simulink model "kick_lowerlimb"  (R2021b)
settings: Solver=FixedStepAuto  StartTime=0.0  StopTime=5  FixedStep=1e-4  RelTol=1e-3  AbsTol=1e-3  EnableMultiTasking=on
values from neighbouring files (symbols this model uses):
  musEnd1 = RN    [runsim.m]
  musEnd2 = RN    [runsim.m]
  musStart1 = -RN    [runsim.m]
  musStart2 = -RN    [runsim.m]
  t1 = 1    [runsim.m]
  t2 = 1.1    [runsim.m]
undefined symbols (not defined in the file or in its folder): intv, param, Param_Mus_MEE, Param_Mus_MEE_hip, Param_Mus_MEE_knee, Param_Mus_MEF, Param_Mus_MEF_hip, Param_Mus_MEF_knee, r, u1, X, Y, Z
libraries: sm_lib x53, Library_mtu_simulink x24, nesl_utility x22
(part 2 of 2)

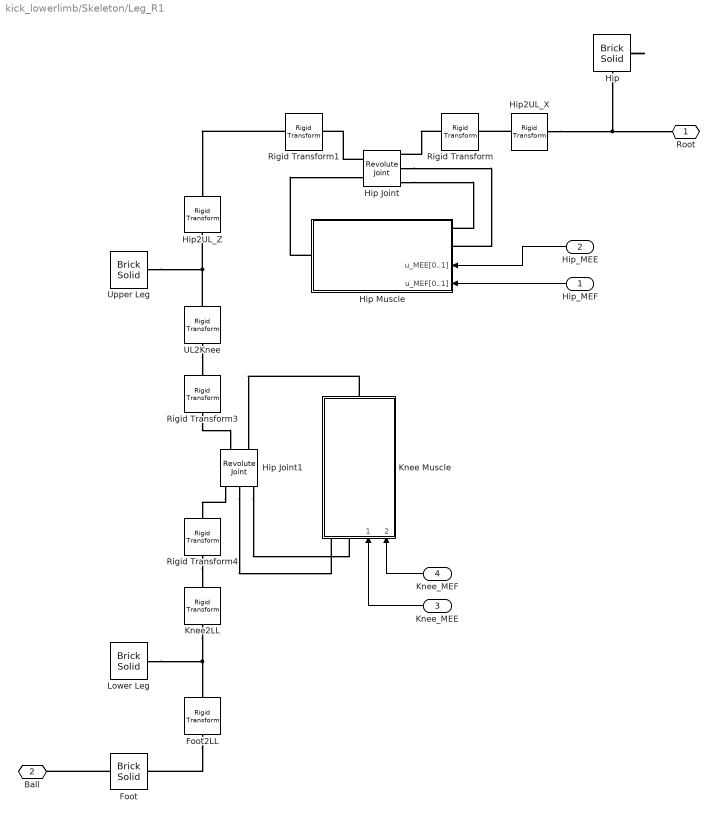
== system kick_lowerlimb/Skeleton/Leg_R1 ==
  Hip_MEF : Inport
  Hip_MEE : Inport  Port=2
  Knee_MEE : Inport  Port=3
  Knee_MEF : Inport  Port=4
  Foot : sm_lib/Body Elements/Brick Solid  GraphicAmbientColor=[0.15 0.15 0.15 1.0]  BasedOnType=Mass  BrickDimensions=param.foot.dim  BrickDimensionUnits=m  CenterOfMass=[0 0 0]  CenterOfMassUnits=m  GraphicDiffuseColor=[0.5 0.5 0.5]  Density=1000  DensityUnits=kg/m^3  DoExposeReferenceFrame=on  GraphicEmissiveColor=[0.0 0.0 0.0 1.0]  ExportEntireGeometry=on  SerializedFrames=<Frames/>  MarkerShape=Sphere  MarkerSize=10  GraphicType=FromGeometry  InertiaType=CalculateFromGeometry  Mass=param.foot.mass  MassUnits=kg  MomentsOfInertia=[1 1 1]  MomentsOfInertiaUnits=kg*m^2  GraphicOpacity=1.0  ProductsOfInertia=[0 0 0]  ProductsOfInertiaUnits=kg*m^2  GraphicShininess=75  GraphicSpecularColor=[0.5 0.5 0.5 1.0]  GraphicVisPropType=SimpleVisualProperties
  Foot2LL : sm_lib/Frames and Transforms/Rigid Transform  TranslationMethod=Cartesian  TranslationStandardOffset=0  TranslationLengthUnit=m  TranslationStandardAxis=+Z  TranslationCartesianOffset=param.ll.pos.foot  TranslationROffset=0  TranslationROffsetUnits=m  TranslationZOffset=0  TranslationZOffsetUnits=m  TranslationThetaOffset=0  TranslationThetaOffsetUnits=deg  RotationMethod=None  RotationAngleUnits=deg  RotationStandardAxis=+Z  RotationAngle=0.0  RotationArbitraryAxis=[0 0 1]  FollAlignAxisA=+X  BaseAlignAxisA=+Y  FollAlignAxisB=+Y  BaseAlignAxisB=+Z  RotationSequenceAxes=FollowerAxes  RotationSequence=XYX  RotationSequenceAngles=[0 0 0]  RotationSequenceAnglesUnits=deg  RotationMatrix=[1 0 0; 0 1 0; 0 0 1]
  Hip : sm_lib/Body Elements/Brick Solid  GraphicAmbientColor=[0.15 0.15 0.15 1.0]  BasedOnType=Mass  BrickDimensions=param.hip.dim  BrickDimensionUnits=m  CenterOfMass=[0 0 0]  CenterOfMassUnits=m  GraphicDiffuseColor=[0.5 0.5 0.5]  Density=1000  DensityUnits=kg/m^3  DoExposeReferenceFrame=on  GraphicEmissiveColor=[0.0 0.0 0.0 1.0]  ExportEntireGeometry=off  SerializedFrames=<Frames/>  MarkerShape=Sphere  MarkerSize=10  GraphicType=FromGeometry  InertiaType=CalculateFromGeometry  Mass=param.hip.mass/2  MassUnits=kg  MomentsOfInertia=[1 1 1]  MomentsOfInertiaUnits=kg*m^2  GraphicOpacity=1.0  ProductsOfInertia=[0 0 0]  ProductsOfInertiaUnits=kg*m^2  GraphicShininess=75  GraphicSpecularColor=[0.5 0.5 0.5 1.0]  GraphicVisPropType=SimpleVisualProperties
  Hip Joint : sm_lib/Joints/Revolute Joint  JointMode=Normal  SenseConstraintForce=off  SenseConstraintForceX=off  SenseConstraintForceY=off  SenseConstraintForceZ=off  SenseConstraintTorque=off  SenseConstraintTorqueX=off  SenseConstraintTorqueY=off  SenseConstraintTorqueZ=off  SenseTotalForce=off  SenseTotalForceX=off  SenseTotalForceY=off  SenseTotalForceZ=off  SenseTotalTorque=off  SenseTotalTorqueX=off  SenseTotalTorqueY=off  SenseTotalTorqueZ=off  CompositeWrenchDir=FollowerOnBase  CompositeWrenchFrame=BaseFrame  EquilibriumPosition=0  EquilibriumPositionUnits=deg  SpringStiffness=0  SpringStiffnessUnits=N*m/deg  DampingCoefficient=0  DampingCoefficientUnits=N*m/(deg/s)  TorqueActuationMode=InputTorque  MotionActuationMode=ComputedMotion  SensePosition=on  SenseVelocity=on  SenseAcceleration=off  SenseTorqueForce=off  SenseLowerLimitTorqueForce=off  SenseUpperLimitTorqueForce=off  LowerLimitSpecify=on  LowerLimitBound=-45  LowerLimitBoundUnits=deg  LowerLimitStiffness=1e4  LowerLimitStiffnessUnits=N*m/deg  LowerLimitDamping=10  LowerLimitDampingUnits=N*m/(deg/s)  LowerLimitTransitionRegionWidth=0.1  LowerLimitTransitionRegionWidthUnits=deg  UpperLimitSpecify=on  UpperLimitBound=90  UpperLimitBoundUnits=deg  UpperLimitStiffness=1e4  UpperLimitStiffnessUnits=N*m/deg  UpperLimitDamping=10  UpperLimitDampingUnits=N*m/(deg/s)  UpperLimitTransitionRegionWidth=0.1  UpperLimitTransitionRegionWidthUnits=deg  PositionTargetSpecify=off  PositionTargetPriority=High  PositionTargetValue=0  PositionTargetValueUnits=deg  VelocityTargetSpecify=off  VelocityTargetPriority=High  VelocityTargetValue=0  VelocityTargetValueUnits=deg/s
  Hip Joint1 : sm_lib/Joints/Revolute Joint  JointMode=Normal  SenseConstraintForce=off  SenseConstraintForceX=off  SenseConstraintForceY=off  SenseConstraintForceZ=off  SenseConstraintTorque=off  SenseConstraintTorqueX=off  SenseConstraintTorqueY=off  SenseConstraintTorqueZ=off  SenseTotalForce=off  SenseTotalForceX=off  SenseTotalForceY=off  SenseTotalForceZ=off  SenseTotalTorque=off  SenseTotalTorqueX=off  SenseTotalTorqueY=off  SenseTotalTorqueZ=off  CompositeWrenchDir=FollowerOnBase  CompositeWrenchFrame=BaseFrame  EquilibriumPosition=0  EquilibriumPositionUnits=deg  SpringStiffness=0  SpringStiffnessUnits=N*m/deg  DampingCoefficient=0  DampingCoefficientUnits=N*m/(deg/s)  TorqueActuationMode=InputTorque  MotionActuationMode=ComputedMotion  SensePosition=on  SenseVelocity=on  SenseAcceleration=off  SenseTorqueForce=off  SenseLowerLimitTorqueForce=off  SenseUpperLimitTorqueForce=off  LowerLimitSpecify=on  LowerLimitBound=-165  LowerLimitBoundUnits=deg  LowerLimitStiffness=1e4  LowerLimitStiffnessUnits=N*m/deg  LowerLimitDamping=10  LowerLimitDampingUnits=N*m/(deg/s)  LowerLimitTransitionRegionWidth=0.1  LowerLimitTransitionRegionWidthUnits=deg  UpperLimitSpecify=on  UpperLimitBound=3  UpperLimitBoundUnits=deg  UpperLimitStiffness=1e4  UpperLimitStiffnessUnits=N*m/deg  UpperLimitDamping=10  UpperLimitDampingUnits=N*m/(deg/s)  UpperLimitTransitionRegionWidth=0.1  UpperLimitTransitionRegionWidthUnits=deg  PositionTargetSpecify=off  PositionTargetPriority=High  PositionTargetValue=0  PositionTargetValueUnits=deg  VelocityTargetSpecify=off  VelocityTargetPriority=High  VelocityTargetValue=0  VelocityTargetValueUnits=deg/s
  Hip Muscle : Subsystem
      settings: PortSchema="{\"entries\":[{\"content\":{\"sides\":[{\"content\":{\"connectorIds\":[\"LConn1\"]},\"type\":\"ConnectorPlacement.EquallySpacedRectSide\",\"uuid\":\"09d485eb-322b-4a2d-b7b4-821800bf0a85\"},{\"content\":{\"connectorIds\":[\"RConn1\",\"RConn2\",\"In1\",\"In2\"],\"side\":\"RIGHT\"},\"type\":\"ConnectorPlacement.EquallySpacedRectSide\",\"uuid\":\"714a60c3-3d51-49b7-818d-6b831f6e3c7a\"},{\"content\":{\"connectorIds\":[],\"side\":\"TOP\"},\"type\":\"ConnectorPlacement.EquallySpacedRectSide\",\"uuid\":\"17f78a34-f772-4722-9987-c43901f4dd6e\"}]},\"type\":\"ConnectorPlacement.EquallySpacedConnector\",\"uuid\":\"fb4f7900-d8a7-436d-9a98-0d4fc98d81d7\"}],\"packageUris\":[\"http://schema.mathworks.com/mf0/Connector/R2020b\"],\"version\":\"1.0\"}"
  Hip2UL_X : sm_lib/Frames and Transforms/Rigid Transform  TranslationMethod=StandardAxis  TranslationStandardOffset=param.hip.pos.ul_x  TranslationLengthUnit=m  TranslationStandardAxis=-X  TranslationCartesianOffset=[0 0 0]  TranslationROffset=0  TranslationROffsetUnits=m  TranslationZOffset=0  TranslationZOffsetUnits=m  TranslationThetaOffset=0  TranslationThetaOffsetUnits=deg  RotationMethod=None  RotationAngleUnits=deg  RotationStandardAxis=+Z  RotationAngle=0.0  RotationArbitraryAxis=[0 0 1]  FollAlignAxisA=+X  BaseAlignAxisA=+Y  FollAlignAxisB=+Y  BaseAlignAxisB=+Z  RotationSequenceAxes=FollowerAxes  RotationSequence=XYX  RotationSequenceAngles=[0 0 0]  RotationSequenceAnglesUnits=deg  RotationMatrix=[1 0 0; 0 1 0; 0 0 1]
  Hip2UL_Z : sm_lib/Frames and Transforms/Rigid Transform  TranslationMethod=StandardAxis  TranslationStandardOffset=param.hip.pos.ul_z  TranslationLengthUnit=m  TranslationStandardAxis=+Z  TranslationCartesianOffset=[0 0 0]  TranslationROffset=0  TranslationROffsetUnits=m  TranslationZOffset=0  TranslationZOffsetUnits=m  TranslationThetaOffset=0  TranslationThetaOffsetUnits=deg  RotationMethod=None  RotationAngleUnits=deg  RotationStandardAxis=+Z  RotationAngle=0.0  RotationArbitraryAxis=[0 0 1]  FollAlignAxisA=+X  BaseAlignAxisA=+Y  FollAlignAxisB=+Y  BaseAlignAxisB=+Z  RotationSequenceAxes=FollowerAxes  RotationSequence=XYX  RotationSequenceAngles=[0 0 0]  RotationSequenceAnglesUnits=deg  RotationMatrix=[1 0 0; 0 1 0; 0 0 1]
  Knee Muscle : Subsystem
      settings: PortSchema="{\"entries\":[{\"content\":{\"sides\":[{\"content\":{\"connectorIds\":[\"LConn1\",\"LConn2\",\"In1\",\"In2\"]},\"type\":\"ConnectorPlacement.EquallySpacedRectSide\",\"uuid\":\"3b044809-3318-4a6d-8aa6-82c54e5fe3cb\"},{\"content\":{\"connectorIds\":[\"RConn1\"],\"side\":\"RIGHT\"},\"type\":\"ConnectorPlacement.EquallySpacedRectSide\",\"uuid\":\"88d11738-42a2-44aa-8fb0-c3ef05d80cd7\"},{\"content\":{\"connectorIds\":[],\"side\":\"TOP\"},\"type\":\"ConnectorPlacement.EquallySpacedRectSide\",\"uuid\":\"f463f2d8-c609-4ddb-8314-070b29d257df\"}]},\"type\":\"ConnectorPlacement.EquallySpacedConnector\",\"uuid\":\"4bbd78e6-9d91-4575-bf34-482a08640315\"}],\"packageUris\":[\"http://schema.mathworks.com/mf0/Connector/R2020b\"],\"version\":\"1.0\"}"
  Knee2LL : sm_lib/Frames and Transforms/Rigid Transform  TranslationMethod=Cartesian  TranslationStandardOffset=0  TranslationLengthUnit=m  TranslationStandardAxis=+Z  TranslationCartesianOffset=param.ll.pos.knee  TranslationROffset=0  TranslationROffsetUnits=m  TranslationZOffset=0  TranslationZOffsetUnits=m  TranslationThetaOffset=0  TranslationThetaOffsetUnits=deg  RotationMethod=None  RotationAngleUnits=deg  RotationStandardAxis=+Z  RotationAngle=0.0  RotationArbitraryAxis=[0 0 1]  FollAlignAxisA=+X  BaseAlignAxisA=+Y  FollAlignAxisB=+Y  BaseAlignAxisB=+Z  RotationSequenceAxes=FollowerAxes  RotationSequence=XYX  RotationSequenceAngles=[0 0 0]  RotationSequenceAnglesUnits=deg  RotationMatrix=[1 0 0; 0 1 0; 0 0 1]
  Lower Leg : sm_lib/Body Elements/Brick Solid  GraphicAmbientColor=[0.15 0.15 0.15 1.0]  BasedOnType=Mass  BrickDimensions=param.ll.dim  BrickDimensionUnits=m  CenterOfMass=[0 0 0]  CenterOfMassUnits=m  GraphicDiffuseColor=[0.2 0.2 1.0]  Density=1000  DensityUnits=kg/m^3  DoExposeReferenceFrame=on  GraphicEmissiveColor=[0.0 0.0 0.0 1.0]  ExportEntireGeometry=off  SerializedFrames=<Frames/>  MarkerShape=Sphere  MarkerSize=10  GraphicType=FromGeometry  InertiaType=CalculateFromGeometry  Mass=param.ll.mass  MassUnits=kg  MomentsOfInertia=[1 1 1]  MomentsOfInertiaUnits=kg*m^2  GraphicOpacity=1.0  ProductsOfInertia=[0 0 0]  ProductsOfInertiaUnits=kg*m^2  GraphicShininess=75  GraphicSpecularColor=[0.5 0.5 0.5 1.0]  GraphicVisPropType=SimpleVisualProperties
  Rigid Transform : sm_lib/Frames and Transforms/Rigid Transform  TranslationMethod=None  TranslationStandardOffset=0  TranslationLengthUnit=m  TranslationStandardAxis=+Z  TranslationCartesianOffset=[0 0 0]  TranslationROffset=0  TranslationROffsetUnits=m  TranslationZOffset=0  TranslationZOffsetUnits=m  TranslationThetaOffset=0  TranslationThetaOffsetUnits=deg  RotationMethod=StandardAxis  RotationAngleUnits=deg  RotationStandardAxis=+Y  RotationAngle=90  RotationArbitraryAxis=[0 0 1]  FollAlignAxisA=+X  BaseAlignAxisA=+Y  FollAlignAxisB=+Y  BaseAlignAxisB=+Z  RotationSequenceAxes=FollowerAxes  RotationSequence=XYX  RotationSequenceAngles=[0 0 0]  RotationSequenceAnglesUnits=deg  RotationMatrix=[1 0 0; 0 1 0; 0 0 1]
  Rigid Transform1 : sm_lib/Frames and Transforms/Rigid Transform  TranslationMethod=None  TranslationStandardOffset=0  TranslationLengthUnit=m  TranslationStandardAxis=+Z  TranslationCartesianOffset=[0 0 0]  TranslationROffset=0  TranslationROffsetUnits=m  TranslationZOffset=0  TranslationZOffsetUnits=m  TranslationThetaOffset=0  TranslationThetaOffsetUnits=deg  RotationMethod=StandardAxis  RotationAngleUnits=deg  RotationStandardAxis=-Y  RotationAngle=90  RotationArbitraryAxis=[0 0 1]  FollAlignAxisA=+X  BaseAlignAxisA=+Y  FollAlignAxisB=+Y  BaseAlignAxisB=+Z  RotationSequenceAxes=FollowerAxes  RotationSequence=XYX  RotationSequenceAngles=[0 0 0]  RotationSequenceAnglesUnits=deg  RotationMatrix=[1 0 0; 0 1 0; 0 0 1]
  Rigid Transform3 : sm_lib/Frames and Transforms/Rigid Transform  TranslationMethod=None  TranslationStandardOffset=0  TranslationLengthUnit=m  TranslationStandardAxis=+Z  TranslationCartesianOffset=[0 0 0]  TranslationROffset=0  TranslationROffsetUnits=m  TranslationZOffset=0  TranslationZOffsetUnits=m  TranslationThetaOffset=0  TranslationThetaOffsetUnits=deg  RotationMethod=StandardAxis  RotationAngleUnits=deg  RotationStandardAxis=+Y  RotationAngle=90  RotationArbitraryAxis=[0 0 1]  FollAlignAxisA=+X  BaseAlignAxisA=+Y  FollAlignAxisB=+Y  BaseAlignAxisB=+Z  RotationSequenceAxes=FollowerAxes  RotationSequence=XYX  RotationSequenceAngles=[0 0 0]  RotationSequenceAnglesUnits=deg  RotationMatrix=[1 0 0; 0 1 0; 0 0 1]
  Rigid Transform4 : sm_lib/Frames and Transforms/Rigid Transform  TranslationMethod=None  TranslationStandardOffset=0  TranslationLengthUnit=m  TranslationStandardAxis=+Z  TranslationCartesianOffset=[0 0 0]  TranslationROffset=0  TranslationROffsetUnits=m  TranslationZOffset=0  TranslationZOffsetUnits=m  TranslationThetaOffset=0  TranslationThetaOffsetUnits=deg  RotationMethod=StandardAxis  RotationAngleUnits=deg  RotationStandardAxis=-Y  RotationAngle=90  RotationArbitraryAxis=[0 0 1]  FollAlignAxisA=+X  BaseAlignAxisA=+Y  FollAlignAxisB=+Y  BaseAlignAxisB=+Z  RotationSequenceAxes=FollowerAxes  RotationSequence=XYX  RotationSequenceAngles=[0 0 0]  RotationSequenceAnglesUnits=deg  RotationMatrix=[1 0 0; 0 1 0; 0 0 1]
  UL2Knee : sm_lib/Frames and Transforms/Rigid Transform  TranslationMethod=Cartesian  TranslationStandardOffset=0  TranslationLengthUnit=m  TranslationStandardAxis=+Z  TranslationCartesianOffset=param.ul.pos.knee  TranslationROffset=0  TranslationROffsetUnits=m  TranslationZOffset=0  TranslationZOffsetUnits=m  TranslationThetaOffset=0  TranslationThetaOffsetUnits=deg  RotationMethod=None  RotationAngleUnits=deg  RotationStandardAxis=+Z  RotationAngle=0.0  RotationArbitraryAxis=[0 0 1]  FollAlignAxisA=+X  BaseAlignAxisA=+Y  FollAlignAxisB=+Y  BaseAlignAxisB=+Z  RotationSequenceAxes=FollowerAxes  RotationSequence=XYX  RotationSequenceAngles=[0 0 0]  RotationSequenceAnglesUnits=deg  RotationMatrix=[1 0 0; 0 1 0; 0 0 1]
  Upper Leg : sm_lib/Body Elements/Brick Solid  GraphicAmbientColor=[0.15 0.15 0.15 1.0]  BasedOnType=Mass  BrickDimensions=param.ul.dim  BrickDimensionUnits=m  CenterOfMass=[0 0 0]  CenterOfMassUnits=m  GraphicDiffuseColor=[0.5 0.5 0.5]  Density=1000  DensityUnits=kg/m^3  DoExposeReferenceFrame=on  GraphicEmissiveColor=[0.0 0.0 0.0 1.0]  ExportEntireGeometry=off  SerializedFrames=<Frames/>  MarkerShape=Sphere  MarkerSize=10  GraphicType=FromGeometry  InertiaType=CalculateFromGeometry  Mass=param.ul.mass  MassUnits=kg  MomentsOfInertia=[1 1 1]  MomentsOfInertiaUnits=kg*m^2  GraphicOpacity=1.0  ProductsOfInertia=[0 0 0]  ProductsOfInertiaUnits=kg*m^2  GraphicShininess=75  GraphicSpecularColor=[0.5 0.5 0.5 1.0]  GraphicVisPropType=SimpleVisualProperties
  Root : PMIOPort  Side=Left
  Ball : PMIOPort  Port=2  Side=Right
  wires:
  Hip_MEF/1 -> Hip Muscle/2(u_MEF[0..1])
  Hip_MEE/1 -> Hip Muscle/1(u_MEE[0..1])
  Knee_MEE/1 -> Knee Muscle/1(u_MEE[0..1])
  Knee_MEF/1 -> Knee Muscle/2(u_MEF[0..1])
  connections:
  Lower Leg/RConn1 -- Knee2LL/RConn1 -- Foot2LL/LConn1
  Foot2LL/RConn1 -- Foot/RConn1
  UL2Knee/LConn1 -- Upper Leg/RConn1 -- Hip2UL_Z/RConn1
  Hip/RConn1 -- Root/RConn1 -- Hip2UL_X/LConn1
  Rigid Transform/LConn1 -- Hip Joint/RConn1
  Hip Joint/LConn1 -- Rigid Transform1/RConn1
  Hip2UL_X/RConn1 -- Rigid Transform/RConn1
  UL2Knee/RConn1 -- Rigid Transform3/LConn1
  Rigid Transform3/RConn1 -- Hip Joint1/LConn1
  Hip Joint1/RConn1 -- Rigid Transform4/LConn1
  Rigid Transform4/RConn1 -- Knee2LL/LConn1
  Foot/LConn1 -- Ball/RConn1
  Hip Joint/RConn2 -- Hip Muscle/RConn2
  Rigid Transform1/LConn1 -- Hip2UL_Z/LConn1
  Hip Joint/RConn3 -- Hip Muscle/RConn1
  Hip Muscle/LConn1 -- Hip Joint/LConn2
  Hip Joint1/RConn2 -- Knee Muscle/LConn1
  Knee Muscle/RConn1 -- Hip Joint1/LConn2
  Hip Joint1/RConn3 -- Knee Muscle/LConn2

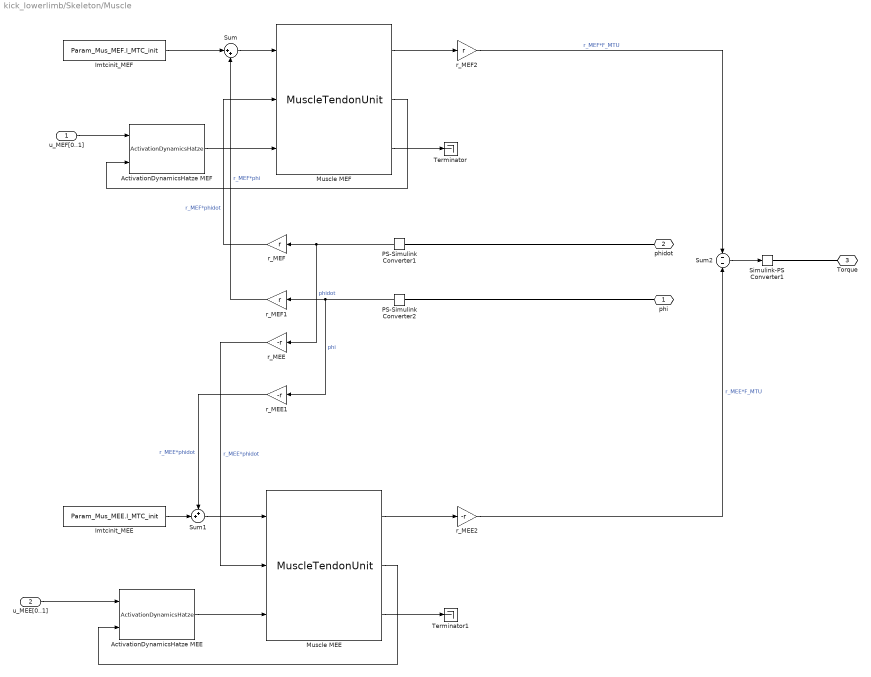
== system kick_lowerlimb/Skeleton/Muscle ==
  u_MEF[0..1] : Inport
  u_MEE[0..1] : Inport  Port=2
  ActivationDynamicsHatze MEE : Library_mtu_simulink/ActivationDynamicsHatze  Act_Param=Param_Mus_MEE.ActDyn  Mus_Param=Param_Mus_MEE
  ActivationDynamicsHatze MEF : Library_mtu_simulink/ActivationDynamicsHatze  Act_Param=Param_Mus_MEF.ActDyn  Mus_Param=Param_Mus_MEF
  Imtcinit_MEE : Constant  Value=Param_Mus_MEE.l_MTC_init
  Imtcinit_MEF : Constant  Value=Param_Mus_MEF.l_MTC_init
  Muscle MEE : Library_mtu_simulink/MuscleTendonUnit  Mus_Param=Param_Mus_MEE
  Muscle MEF : Library_mtu_simulink/MuscleTendonUnit  Mus_Param=Param_Mus_MEF
  PS-Simulink Converter1 : nesl_utility/PS-Simulink Converter  PhysicalDomain=network_engine_domain  SubClassName=ps_output  LeftPortType=input  RightPortType=output  PseudoPeriodic=off  Frequencies=[]  Unit=inherit  AffineConversion=off
      settings: SourceProductBaseCode=PW,SS
  PS-Simulink Converter2 : nesl_utility/PS-Simulink Converter  PhysicalDomain=network_engine_domain  SubClassName=ps_output  LeftPortType=input  RightPortType=output  PseudoPeriodic=off  Frequencies=[]  Unit=inherit  AffineConversion=off
      settings: SourceProductBaseCode=PW,SS
  Simulink-PS Converter1 : nesl_utility/Simulink-PS Converter  PhysicalDomain=network_engine_domain  SubClassName=ps_input  LeftPortType=input  RightPortType=output  PseudoPeriodic=off  Frequencies=[]  NoiseDistribution=none  NoiseParameters=[]  Unit=1  AffineConversion=off  FilteringAndDerivatives=provide  SimscapeFilterOrder=1  InputFilterTimeConstant=0.001  UdotUserProvided=0
      settings: SourceProductBaseCode=PW,SS
  Sum : Sum  Inputs=|++
  Sum1 : Sum  Inputs=++|
  Sum2 : Sum  Inputs=--
  Terminator : Terminator
  Terminator1 : Terminator
  r_MEE : Gain  Gain=-r
  r_MEE1 : Gain  Gain=-r
  r_MEE2 : Gain  Gain=-r
  r_MEF : Gain  Gain=r
  r_MEF1 : Gain  Gain=r
  r_MEF2 : Gain  Gain=r
  phi : PMIOPort  Side=Left
  phidot : PMIOPort  Port=2  Side=Left
  Torque : PMIOPort  Port=3  Side=Right
  wires:
  r_MEE/1 -> Muscle MEE/2  "r_MEE*phidot"
  Imtcinit_MEE/1 -> Sum1/2
  ActivationDynamicsHatze MEF/1 -> Muscle MEF/3
  PS-Simulink Converter2/1 -> r_MEF1/1, r_MEE1/1  "phi"
  r_MEE2/1 -> Sum2/2  "r_MEE*F_MTU"
  u_MEF[0..1]/1 -> ActivationDynamicsHatze MEF/1
  Muscle MEF/3 -> Terminator/1
  r_MEF/1 -> Muscle MEF/2  "r_MEF*phidot"
  Sum/1 -> Muscle MEF/1
  Muscle MEE/1 -> r_MEE2/1
  r_MEE1/1 -> Sum1/1  "r_MEE*phidot"
  r_MEF1/1 -> Sum/2  "r_MEF*phi"
  u_MEE[0..1]/1 -> ActivationDynamicsHatze MEE/1
  Sum2/1 -> Simulink-PS Converter1/1
  Sum1/1 -> Muscle MEE/1
  Imtcinit_MEF/1 -> Sum/1
  PS-Simulink Converter1/1 -> r_MEF/1, r_MEE/1  "phidot"
  ActivationDynamicsHatze MEE/1 -> Muscle MEE/3
  Muscle MEE/2 -> ActivationDynamicsHatze MEE/2
  Muscle MEE/3 -> Terminator1/1
  Muscle MEF/1 -> r_MEF2/1
  Muscle MEF/2 -> ActivationDynamicsHatze MEF/2
  r_MEF2/1 -> Sum2/1  "r_MEF*F_MTU"
  connections:
  Torque/RConn1 -- Simulink-PS Converter1/RConn1
  PS-Simulink Converter2/LConn1 -- phi/RConn1
  PS-Simulink Converter1/LConn1 -- phidot/RConn1

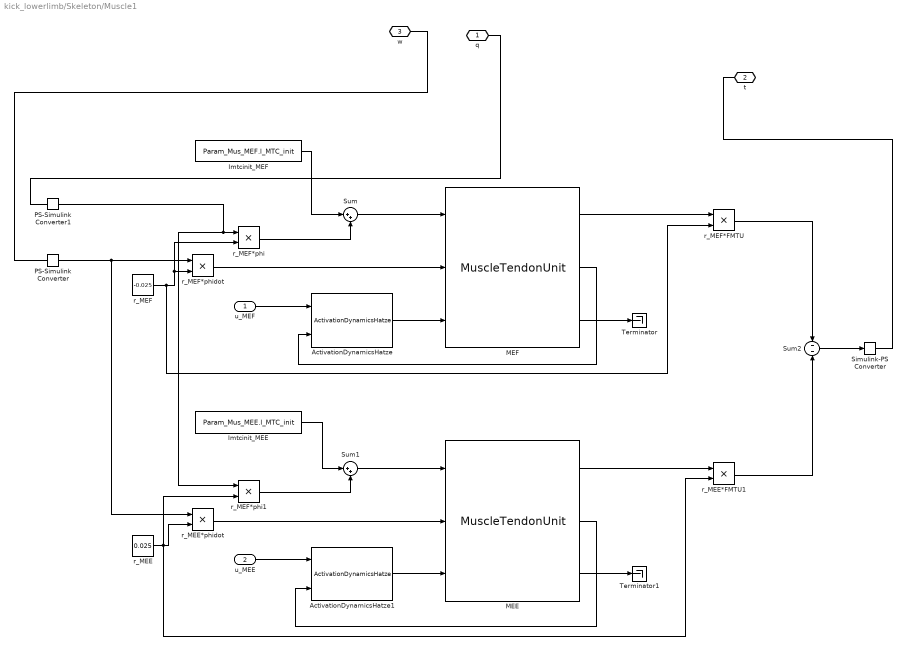
== system kick_lowerlimb/Skeleton/Muscle1 ==
  u_MEF : Inport
  u_MEE : Inport  Port=2
  ActivationDynamicsHatze : Library_mtu_simulink/ActivationDynamicsHatze  Act_Param=Param_Mus_MEF.ActDyn  Mus_Param=Param_Mus_MEF
  ActivationDynamicsHatze1 : Library_mtu_simulink/ActivationDynamicsHatze  Act_Param=Param_Mus_MEE.ActDyn  Mus_Param=Param_Mus_MEE
  Imtcinit_MEE : Constant  Value=Param_Mus_MEE.l_MTC_init
  Imtcinit_MEF : Constant  Value=Param_Mus_MEF.l_MTC_init
  MEE : Library_mtu_simulink/MuscleTendonUnit  Mus_Param=Param_Mus_MEE
  MEF : Library_mtu_simulink/MuscleTendonUnit  Mus_Param=Param_Mus_MEF
  PS-Simulink Converter : nesl_utility/PS-Simulink Converter  PhysicalDomain=network_engine_domain  SubClassName=ps_output  LeftPortType=input  RightPortType=output  PseudoPeriodic=off  Frequencies=[]  Unit=inherit  AffineConversion=off
      settings: SourceProductBaseCode=PW,SS
  PS-Simulink Converter1 : nesl_utility/PS-Simulink Converter  PhysicalDomain=network_engine_domain  SubClassName=ps_output  LeftPortType=input  RightPortType=output  PseudoPeriodic=off  Frequencies=[]  Unit=inherit  AffineConversion=off
      settings: SourceProductBaseCode=PW,SS
  Simulink-PS Converter : nesl_utility/Simulink-PS Converter  PhysicalDomain=network_engine_domain  SubClassName=ps_input  LeftPortType=input  RightPortType=output  PseudoPeriodic=off  Frequencies=[]  NoiseDistribution=none  NoiseParameters=[]  Unit=1  AffineConversion=off  FilteringAndDerivatives=provide  SimscapeFilterOrder=1  InputFilterTimeConstant=0.001  UdotUserProvided=0
      settings: SourceProductBaseCode=PW,SS
  Sum : Sum  Inputs=|++
  Sum1 : Sum  Inputs=|++
  Sum2 : Sum  Inputs=--
  Terminator : Terminator
  Terminator1 : Terminator
  r_MEE : Constant  Value=0.025
  r_MEE*FMTU1 : Product
  r_MEE*phidot : Product
  r_MEF : Constant  Value=-0.025
  r_MEF*FMTU : Product
  r_MEF*phi : Product
  r_MEF*phi1 : Product
  r_MEF*phidot : Product
  q : PMIOPort  Side=Left
  t : PMIOPort  Port=2  Side=Right
  w : PMIOPort  Port=3  Side=Left
  wires:
  r_MEE*FMTU1/1 -> Sum2/2
  r_MEF*FMTU/1 -> Sum2/1
  MEF/3 -> Terminator/1
  r_MEE*phidot/1 -> MEE/2
  Sum2/1 -> Simulink-PS Converter/1
  PS-Simulink Converter1/1 -> r_MEF*phi1/1, r_MEF*phi/1
  PS-Simulink Converter/1 -> r_MEE*phidot/1, r_MEF*phidot/1
  r_MEE/1 -> r_MEE*FMTU1/2, r_MEF*phi1/2, r_MEE*phidot/2
  MEE/2 -> ActivationDynamicsHatze1/2
  Sum/1 -> MEF/1
  r_MEF*phi1/1 -> Sum1/2
  Imtcinit_MEE/1 -> Sum1/1
  MEE/3 -> Terminator1/1
  Imtcinit_MEF/1 -> Sum/1
  u_MEE/1 -> ActivationDynamicsHatze1/1
  r_MEF/1 -> r_MEF*FMTU/2, r_MEF*phi/2, r_MEF*phidot/2
  u_MEF/1 -> ActivationDynamicsHatze/1
  Sum1/1 -> MEE/1
  MEF/1 -> r_MEF*FMTU/1
  ActivationDynamicsHatze1/1 -> MEE/3
  r_MEF*phidot/1 -> MEF/2
  r_MEF*phi/1 -> Sum/2
  MEE/1 -> r_MEE*FMTU1/1
  MEF/2 -> ActivationDynamicsHatze/2
  ActivationDynamicsHatze/1 -> MEF/3
  connections:
  PS-Simulink Converter1/LConn1 -- q/RConn1
  Simulink-PS Converter/RConn1 -- t/RConn1
  PS-Simulink Converter/LConn1 -- w/RConn1

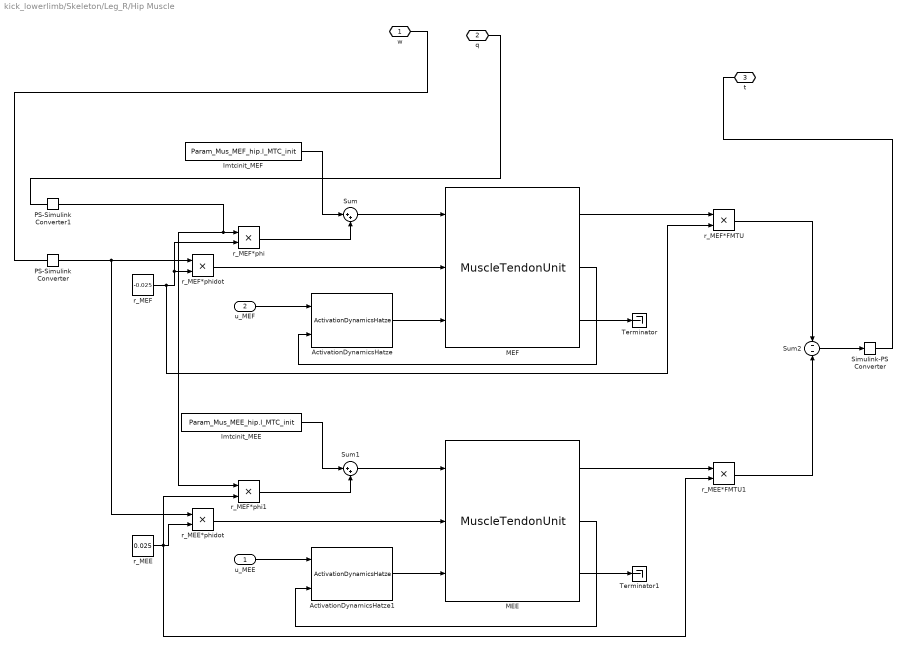
== system kick_lowerlimb/Skeleton/Leg_R/Hip Muscle ==
  u_MEE : Inport
  u_MEF : Inport  Port=2
  ActivationDynamicsHatze : Library_mtu_simulink/ActivationDynamicsHatze  Act_Param=Param_Mus_MEF_hip.ActDyn  Mus_Param=Param_Mus_MEF_hip
  ActivationDynamicsHatze1 : Library_mtu_simulink/ActivationDynamicsHatze  Act_Param=Param_Mus_MEE_hip.ActDyn  Mus_Param=Param_Mus_MEE_hip
  Imtcinit_MEE : Constant  Value=Param_Mus_MEE_hip.l_MTC_init
  Imtcinit_MEF : Constant  Value=Param_Mus_MEF_hip.l_MTC_init
  MEE : Library_mtu_simulink/MuscleTendonUnit  Mus_Param=Param_Mus_MEE_hip
  MEF : Library_mtu_simulink/MuscleTendonUnit  Mus_Param=Param_Mus_MEF_hip
  PS-Simulink Converter : nesl_utility/PS-Simulink Converter  PhysicalDomain=network_engine_domain  SubClassName=ps_output  LeftPortType=input  RightPortType=output  PseudoPeriodic=off  Frequencies=[]  Unit=inherit  AffineConversion=off
      settings: SourceProductBaseCode=PW,SS
  PS-Simulink Converter1 : nesl_utility/PS-Simulink Converter  PhysicalDomain=network_engine_domain  SubClassName=ps_output  LeftPortType=input  RightPortType=output  PseudoPeriodic=off  Frequencies=[]  Unit=inherit  AffineConversion=off
      settings: SourceProductBaseCode=PW,SS
  Simulink-PS Converter : nesl_utility/Simulink-PS Converter  PhysicalDomain=network_engine_domain  SubClassName=ps_input  LeftPortType=input  RightPortType=output  PseudoPeriodic=off  Frequencies=[]  NoiseDistribution=none  NoiseParameters=[]  Unit=1  AffineConversion=off  FilteringAndDerivatives=provide  SimscapeFilterOrder=1  InputFilterTimeConstant=0.001  UdotUserProvided=0
      settings: SourceProductBaseCode=PW,SS
  Sum : Sum  Inputs=|++
  Sum1 : Sum  Inputs=|++
  Sum2 : Sum  Inputs=--
  Terminator : Terminator
  Terminator1 : Terminator
  r_MEE : Constant  Value=0.025
  r_MEE*FMTU1 : Product
  r_MEE*phidot : Product
  r_MEF : Constant  Value=-0.025
  r_MEF*FMTU : Product
  r_MEF*phi : Product
  r_MEF*phi1 : Product
  r_MEF*phidot : Product
  w : PMIOPort  Side=Left
  q : PMIOPort  Port=2  Side=Left
  t : PMIOPort  Port=3  Side=Right
  wires:
  r_MEE*FMTU1/1 -> Sum2/2
  r_MEF*FMTU/1 -> Sum2/1
  MEF/3 -> Terminator/1
  r_MEE*phidot/1 -> MEE/2
  Sum2/1 -> Simulink-PS Converter/1
  PS-Simulink Converter1/1 -> r_MEF*phi1/1, r_MEF*phi/1
  PS-Simulink Converter/1 -> r_MEE*phidot/1, r_MEF*phidot/1
  r_MEE/1 -> r_MEE*FMTU1/2, r_MEF*phi1/2, r_MEE*phidot/2
  MEE/2 -> ActivationDynamicsHatze1/2
  Sum/1 -> MEF/1
  r_MEF*phi1/1 -> Sum1/2
  Imtcinit_MEE/1 -> Sum1/1
  MEE/3 -> Terminator1/1
  Imtcinit_MEF/1 -> Sum/1
  u_MEE/1 -> ActivationDynamicsHatze1/1
  r_MEF/1 -> r_MEF*FMTU/2, r_MEF*phi/2, r_MEF*phidot/2
  u_MEF/1 -> ActivationDynamicsHatze/1
  Sum1/1 -> MEE/1
  MEF/1 -> r_MEF*FMTU/1
  ActivationDynamicsHatze1/1 -> MEE/3
  r_MEF*phidot/1 -> MEF/2
  r_MEF*phi/1 -> Sum/2
  MEE/1 -> r_MEE*FMTU1/1
  MEF/2 -> ActivationDynamicsHatze/2
  ActivationDynamicsHatze/1 -> MEF/3
  connections:
  PS-Simulink Converter1/LConn1 -- q/RConn1
  Simulink-PS Converter/RConn1 -- t/RConn1
  PS-Simulink Converter/LConn1 -- w/RConn1

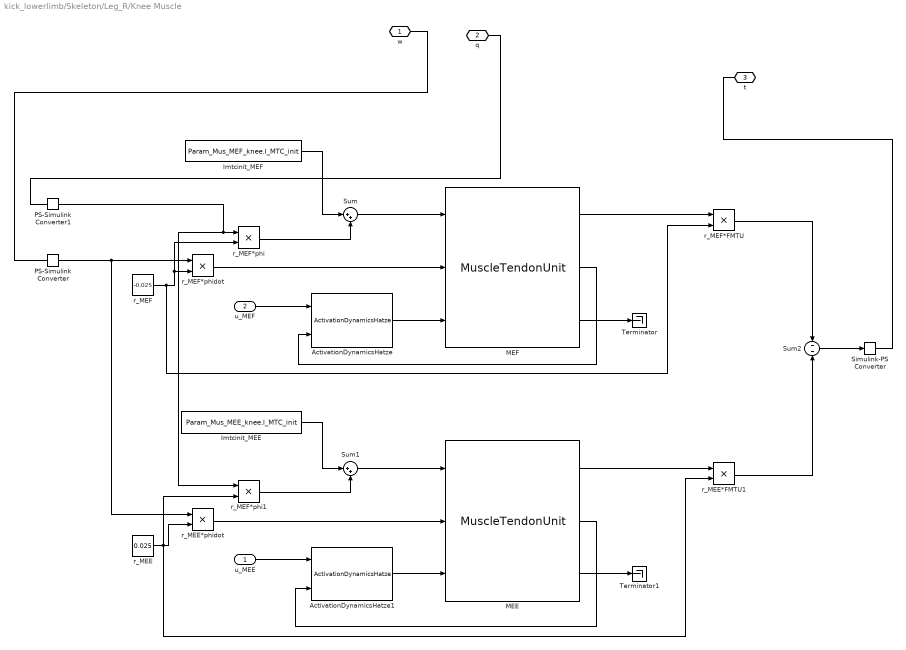
== system kick_lowerlimb/Skeleton/Leg_R/Knee Muscle ==
  u_MEE : Inport
  u_MEF : Inport  Port=2
  ActivationDynamicsHatze : Library_mtu_simulink/ActivationDynamicsHatze  Act_Param=Param_Mus_MEF_knee.ActDyn  Mus_Param=Param_Mus_MEF_knee
  ActivationDynamicsHatze1 : Library_mtu_simulink/ActivationDynamicsHatze  Act_Param=Param_Mus_MEE_knee.ActDyn  Mus_Param=Param_Mus_MEE_knee
  Imtcinit_MEE : Constant  Value=Param_Mus_MEE_knee.l_MTC_init
  Imtcinit_MEF : Constant  Value=Param_Mus_MEF_knee.l_MTC_init
  MEE : Library_mtu_simulink/MuscleTendonUnit  Mus_Param=Param_Mus_MEE_knee
  MEF : Library_mtu_simulink/MuscleTendonUnit  Mus_Param=Param_Mus_MEF_knee
  PS-Simulink Converter : nesl_utility/PS-Simulink Converter  PhysicalDomain=network_engine_domain  SubClassName=ps_output  LeftPortType=input  RightPortType=output  PseudoPeriodic=off  Frequencies=[]  Unit=inherit  AffineConversion=off
      settings: SourceProductBaseCode=PW,SS
  PS-Simulink Converter1 : nesl_utility/PS-Simulink Converter  PhysicalDomain=network_engine_domain  SubClassName=ps_output  LeftPortType=input  RightPortType=output  PseudoPeriodic=off  Frequencies=[]  Unit=inherit  AffineConversion=off
      settings: SourceProductBaseCode=PW,SS
  Simulink-PS Converter : nesl_utility/Simulink-PS Converter  PhysicalDomain=network_engine_domain  SubClassName=ps_input  LeftPortType=input  RightPortType=output  PseudoPeriodic=off  Frequencies=[]  NoiseDistribution=none  NoiseParameters=[]  Unit=1  AffineConversion=off  FilteringAndDerivatives=provide  SimscapeFilterOrder=1  InputFilterTimeConstant=0.001  UdotUserProvided=0
      settings: SourceProductBaseCode=PW,SS
  Sum : Sum  Inputs=|++
  Sum1 : Sum  Inputs=|++
  Sum2 : Sum  Inputs=--
  Terminator : Terminator
  Terminator1 : Terminator
  r_MEE : Constant  Value=0.025
  r_MEE*FMTU1 : Product
  r_MEE*phidot : Product
  r_MEF : Constant  Value=-0.025
  r_MEF*FMTU : Product
  r_MEF*phi : Product
  r_MEF*phi1 : Product
  r_MEF*phidot : Product
  w : PMIOPort  Side=Left
  q : PMIOPort  Port=2  Side=Left
  t : PMIOPort  Port=3  Side=Right
  wires:
  r_MEE*FMTU1/1 -> Sum2/2
  r_MEF*FMTU/1 -> Sum2/1
  MEF/3 -> Terminator/1
  r_MEE*phidot/1 -> MEE/2
  Sum2/1 -> Simulink-PS Converter/1
  PS-Simulink Converter1/1 -> r_MEF*phi1/1, r_MEF*phi/1
  PS-Simulink Converter/1 -> r_MEE*phidot/1, r_MEF*phidot/1
  r_MEE/1 -> r_MEE*FMTU1/2, r_MEF*phi1/2, r_MEE*phidot/2
  MEE/2 -> ActivationDynamicsHatze1/2
  Sum/1 -> MEF/1
  r_MEF*phi1/1 -> Sum1/2
  Imtcinit_MEE/1 -> Sum1/1
  MEE/3 -> Terminator1/1
  Imtcinit_MEF/1 -> Sum/1
  u_MEE/1 -> ActivationDynamicsHatze1/1
  r_MEF/1 -> r_MEF*FMTU/2, r_MEF*phi/2, r_MEF*phidot/2
  u_MEF/1 -> ActivationDynamicsHatze/1
  Sum1/1 -> MEE/1
  MEF/1 -> r_MEF*FMTU/1
  ActivationDynamicsHatze1/1 -> MEE/3
  r_MEF*phidot/1 -> MEF/2
  r_MEF*phi/1 -> Sum/2
  MEE/1 -> r_MEE*FMTU1/1
  MEF/2 -> ActivationDynamicsHatze/2
  ActivationDynamicsHatze/1 -> MEF/3
  connections:
  PS-Simulink Converter1/LConn1 -- q/RConn1
  Simulink-PS Converter/RConn1 -- t/RConn1
  PS-Simulink Converter/LConn1 -- w/RConn1

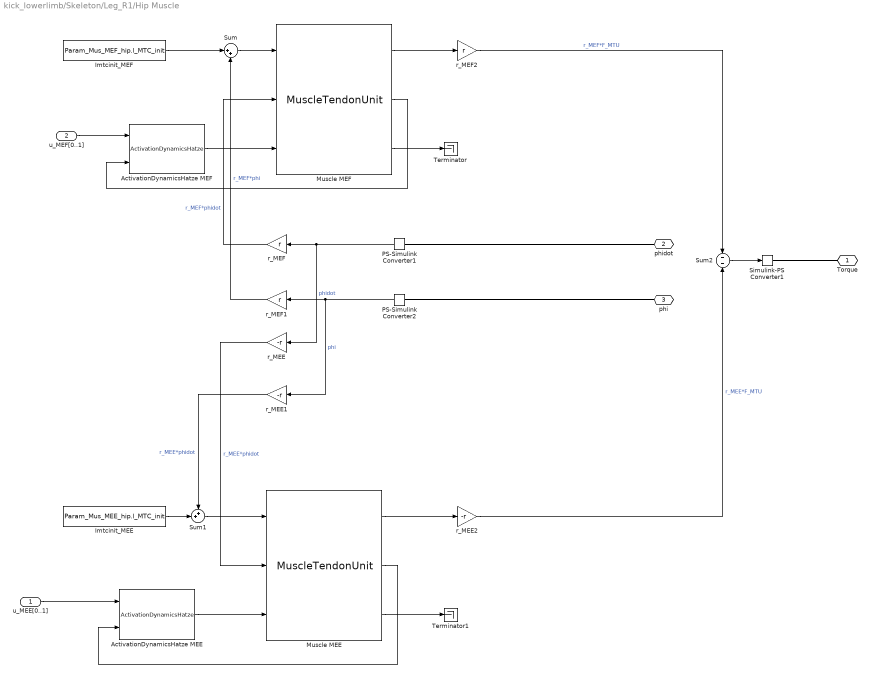
== system kick_lowerlimb/Skeleton/Leg_R1/Hip Muscle ==
  u_MEE[0..1] : Inport
  u_MEF[0..1] : Inport  Port=2
  ActivationDynamicsHatze MEE : Library_mtu_simulink/ActivationDynamicsHatze  Act_Param=Param_Mus_MEE_hip.ActDyn  Mus_Param=Param_Mus_MEE_hip
  ActivationDynamicsHatze MEF : Library_mtu_simulink/ActivationDynamicsHatze  Act_Param=Param_Mus_MEF_hip.ActDyn  Mus_Param=Param_Mus_MEF_hip
  Imtcinit_MEE : Constant  Value=Param_Mus_MEE_hip.l_MTC_init
  Imtcinit_MEF : Constant  Value=Param_Mus_MEF_hip.l_MTC_init
  Muscle MEE : Library_mtu_simulink/MuscleTendonUnit  Mus_Param=Param_Mus_MEE_hip
  Muscle MEF : Library_mtu_simulink/MuscleTendonUnit  Mus_Param=Param_Mus_MEF_hip
  PS-Simulink Converter1 : nesl_utility/PS-Simulink Converter  PhysicalDomain=network_engine_domain  SubClassName=ps_output  LeftPortType=input  RightPortType=output  PseudoPeriodic=off  Frequencies=[]  Unit=inherit  AffineConversion=off
      settings: SourceProductBaseCode=PW,SS
  PS-Simulink Converter2 : nesl_utility/PS-Simulink Converter  PhysicalDomain=network_engine_domain  SubClassName=ps_output  LeftPortType=input  RightPortType=output  PseudoPeriodic=off  Frequencies=[]  Unit=inherit  AffineConversion=off
      settings: SourceProductBaseCode=PW,SS
  Simulink-PS Converter1 : nesl_utility/Simulink-PS Converter  PhysicalDomain=network_engine_domain  SubClassName=ps_input  LeftPortType=input  RightPortType=output  PseudoPeriodic=off  Frequencies=[]  NoiseDistribution=none  NoiseParameters=[]  Unit=1  AffineConversion=off  FilteringAndDerivatives=provide  SimscapeFilterOrder=1  InputFilterTimeConstant=0.001  UdotUserProvided=0
      settings: SourceProductBaseCode=PW,SS
  Sum : Sum  Inputs=|++
  Sum1 : Sum  Inputs=++|
  Sum2 : Sum  Inputs=--
  Terminator : Terminator
  Terminator1 : Terminator
  r_MEE : Gain  Gain=-r
  r_MEE1 : Gain  Gain=-r
  r_MEE2 : Gain  Gain=-r
  r_MEF : Gain  Gain=r
  r_MEF1 : Gain  Gain=r
  r_MEF2 : Gain  Gain=r
  Torque : PMIOPort  Side=Left
  phidot : PMIOPort  Port=2  Side=Right
  phi : PMIOPort  Port=3  Side=Right
  wires:
  r_MEE/1 -> Muscle MEE/2  "r_MEE*phidot"
  Imtcinit_MEE/1 -> Sum1/2
  ActivationDynamicsHatze MEF/1 -> Muscle MEF/3
  PS-Simulink Converter2/1 -> r_MEF1/1, r_MEE1/1  "phi"
  r_MEE2/1 -> Sum2/2  "r_MEE*F_MTU"
  u_MEF[0..1]/1 -> ActivationDynamicsHatze MEF/1
  Muscle MEF/3 -> Terminator/1
  r_MEF/1 -> Muscle MEF/2  "r_MEF*phidot"
  Sum/1 -> Muscle MEF/1
  Muscle MEE/1 -> r_MEE2/1
  r_MEE1/1 -> Sum1/1  "r_MEE*phidot"
  r_MEF1/1 -> Sum/2  "r_MEF*phi"
  u_MEE[0..1]/1 -> ActivationDynamicsHatze MEE/1
  Sum2/1 -> Simulink-PS Converter1/1
  Sum1/1 -> Muscle MEE/1
  Imtcinit_MEF/1 -> Sum/1
  PS-Simulink Converter1/1 -> r_MEF/1, r_MEE/1  "phidot"
  ActivationDynamicsHatze MEE/1 -> Muscle MEE/3
  Muscle MEE/2 -> ActivationDynamicsHatze MEE/2
  Muscle MEE/3 -> Terminator1/1
  Muscle MEF/1 -> r_MEF2/1
  Muscle MEF/2 -> ActivationDynamicsHatze MEF/2
  r_MEF2/1 -> Sum2/1  "r_MEF*F_MTU"
  connections:
  Torque/RConn1 -- Simulink-PS Converter1/RConn1
  PS-Simulink Converter2/LConn1 -- phi/RConn1
  PS-Simulink Converter1/LConn1 -- phidot/RConn1

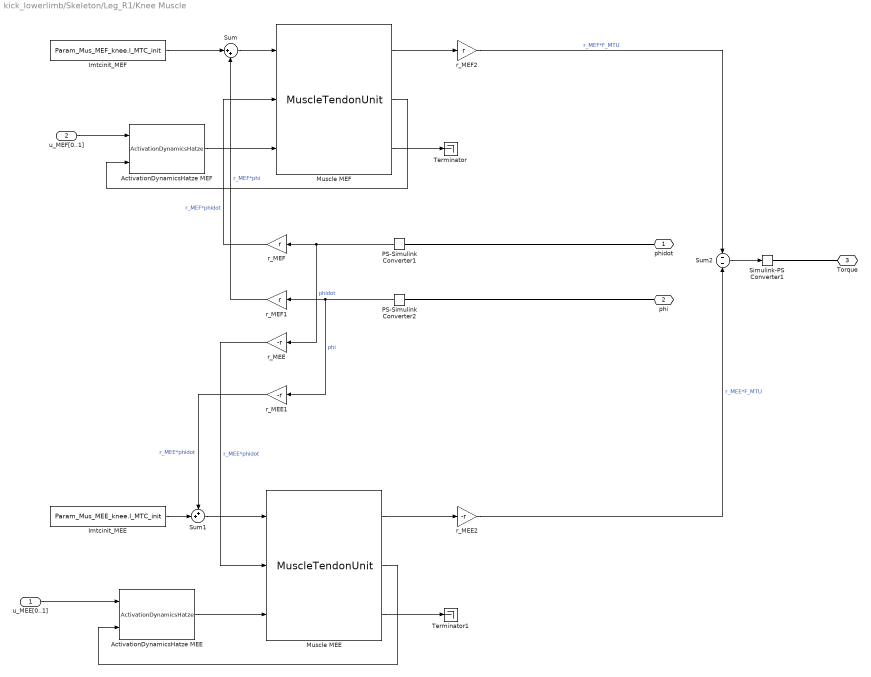
== system kick_lowerlimb/Skeleton/Leg_R1/Knee Muscle ==
  u_MEE[0..1] : Inport
  u_MEF[0..1] : Inport  Port=2
  ActivationDynamicsHatze MEE : Library_mtu_simulink/ActivationDynamicsHatze  Act_Param=Param_Mus_MEE_knee.ActDyn  Mus_Param=Param_Mus_MEE_knee
  ActivationDynamicsHatze MEF : Library_mtu_simulink/ActivationDynamicsHatze  Act_Param=Param_Mus_MEF_knee.ActDyn  Mus_Param=Param_Mus_MEF_knee
  Imtcinit_MEE : Constant  Value=Param_Mus_MEE_knee.l_MTC_init
  Imtcinit_MEF : Constant  Value=Param_Mus_MEF_knee.l_MTC_init
  Muscle MEE : Library_mtu_simulink/MuscleTendonUnit  Mus_Param=Param_Mus_MEE_knee
  Muscle MEF : Library_mtu_simulink/MuscleTendonUnit  Mus_Param=Param_Mus_MEF_knee
  PS-Simulink Converter1 : nesl_utility/PS-Simulink Converter  PhysicalDomain=network_engine_domain  SubClassName=ps_output  LeftPortType=input  RightPortType=output  PseudoPeriodic=off  Frequencies=[]  Unit=inherit  AffineConversion=off
      settings: SourceProductBaseCode=PW,SS
  PS-Simulink Converter2 : nesl_utility/PS-Simulink Converter  PhysicalDomain=network_engine_domain  SubClassName=ps_output  LeftPortType=input  RightPortType=output  PseudoPeriodic=off  Frequencies=[]  Unit=inherit  AffineConversion=off
      settings: SourceProductBaseCode=PW,SS
  Simulink-PS Converter1 : nesl_utility/Simulink-PS Converter  PhysicalDomain=network_engine_domain  SubClassName=ps_input  LeftPortType=input  RightPortType=output  PseudoPeriodic=off  Frequencies=[]  NoiseDistribution=none  NoiseParameters=[]  Unit=1  AffineConversion=off  FilteringAndDerivatives=provide  SimscapeFilterOrder=1  InputFilterTimeConstant=0.001  UdotUserProvided=0
      settings: SourceProductBaseCode=PW,SS
  Sum : Sum  Inputs=|++
  Sum1 : Sum  Inputs=++|
  Sum2 : Sum  Inputs=--
  Terminator : Terminator
  Terminator1 : Terminator
  r_MEE : Gain  Gain=-r
  r_MEE1 : Gain  Gain=-r
  r_MEE2 : Gain  Gain=-r
  r_MEF : Gain  Gain=r
  r_MEF1 : Gain  Gain=r
  r_MEF2 : Gain  Gain=r
  phidot : PMIOPort  Side=Left
  phi : PMIOPort  Port=2  Side=Left
  Torque : PMIOPort  Port=3  Side=Right
  wires:
  r_MEE/1 -> Muscle MEE/2  "r_MEE*phidot"
  Imtcinit_MEE/1 -> Sum1/2
  ActivationDynamicsHatze MEF/1 -> Muscle MEF/3
  PS-Simulink Converter2/1 -> r_MEF1/1, r_MEE1/1  "phi"
  r_MEE2/1 -> Sum2/2  "r_MEE*F_MTU"
  u_MEF[0..1]/1 -> ActivationDynamicsHatze MEF/1
  Muscle MEF/3 -> Terminator/1
  r_MEF/1 -> Muscle MEF/2  "r_MEF*phidot"
  Sum/1 -> Muscle MEF/1
  Muscle MEE/1 -> r_MEE2/1
  r_MEE1/1 -> Sum1/1  "r_MEE*phidot"
  r_MEF1/1 -> Sum/2  "r_MEF*phi"
  u_MEE[0..1]/1 -> ActivationDynamicsHatze MEE/1
  Sum2/1 -> Simulink-PS Converter1/1
  Sum1/1 -> Muscle MEE/1
  Imtcinit_MEF/1 -> Sum/1
  PS-Simulink Converter1/1 -> r_MEF/1, r_MEE/1  "phidot"
  ActivationDynamicsHatze MEE/1 -> Muscle MEE/3
  Muscle MEE/2 -> ActivationDynamicsHatze MEE/2
  Muscle MEE/3 -> Terminator1/1
  Muscle MEF/1 -> r_MEF2/1
  Muscle MEF/2 -> ActivationDynamicsHatze MEF/2
  r_MEF2/1 -> Sum2/1  "r_MEF*F_MTU"
  connections:
  Torque/RConn1 -- Simulink-PS Converter1/RConn1
  PS-Simulink Converter2/LConn1 -- phi/RConn1
  PS-Simulink Converter1/LConn1 -- phidot/RConn1
